simulink model "ReplayPosFilter"  (Simulink 7.8)
settings: Solver=FixedStepDiscrete  StartTime=0.0  StopTime=time(end)  FixedStep=.01  RelTol=1e-3
values from neighbouring files (symbols this model uses):
  apSampleTime = 0.01    [Load_Replay.m]    (also in loadReplayMay2013.m; loadTuneRollReplay_May2013.m; replayFlight.m)
  barAdjust = -6    [replayFlight.m]
  baroCutoff = 0.2/(2*pi)    (= 0.0318309886184)    [replayFlight.m]
  baroCutTemp = -50.0    (= -50)    [replayFlight.m]
  baroOffset = P(2)    [replayFlight.m]
  baroScale = P(1)    [replayFlight.m]
  barTGain1 = -0.0102663    [replayFlight.m]
  barTGain2 = 0.0207608    [replayFlight.m]
  barTMean1 = -161.3    [replayFlight.m]
  barTMean2 = 347.23    [replayFlight.m]
  baseHeight = GS_location(1)    [Load_Replay.m]    (also in loadReplayMay2013.m; loadTuneRollReplay_May2013.m; replayFlight.m = 225)
  baseTemp = 288.215    [GetBaroAlt.m]    (also in replayFlight.m)
  GS_location = [180 36.9898376464844 -122.051963806152]    [Load_Replay.m]    (also in loadReplayMay2013.m; loadTuneRollReplay_May2013.m; replayFlight.m = [0 36.9898376464844 -122.051963806152])
  lapseRate = -0.00198122    [replayFlight.m]
  maxDynPressure = 3000    [replayFlight.m]
  pitAdjust = -41    [replayFlight.m]
  pitCutTemp = -130.0    (= -130)    [replayFlight.m]
  pitotOffset = -1083.881038056753    (= -1083.88103806)    [replayFlight.m]
  pitotScale = 1.213292590242    (= 1.21329259024)    [replayFlight.m]
  pitTGain1 = -0.0552923    [replayFlight.m]
  pitTGain2 = -0.0950433    [replayFlight.m]
  pitTMean1 = -202.93    [replayFlight.m]
  pitTMean2 = 293.053    [replayFlight.m]
  pressureSensorCutoff = 5    [replayFlight.m]
  TData = 0.01    [Load_Replay.m]    (also in loadReplayMay2013.m; loadTuneRollReplay_May2013.m)
  Ts = apSampleTime    (= 0.01)    [Load_Replay.m]    (also in loadReplayMay2013.m; loadTuneRollReplay_May2013.m)
undefined symbols (not defined in the file or in its folder): gaind, getGSLocation, Init_onlyOnce, Init_Reset, polesd, y1, zerosd
libraries: simulink x6, aerolibconvert2 x2, SLUGS_Library x2, dsPICdrivers x1
(part 1 of 2)
settings Model: Creator=Administrator  LastModifiedBy=User
settings OptimizationCC: InitFltsAndDblsToZero=on
settings DebuggingCC: SaveWithParameterizedLinksMsg=none  FcnCallInpInsideContextMsg=Use local settings  StrictBusMsg=Warning
settings SFSimCC: SimParseCustomCode=off
settings GRTTargetCC: TargetFcnLib=ansi_tfl_tmw.mat

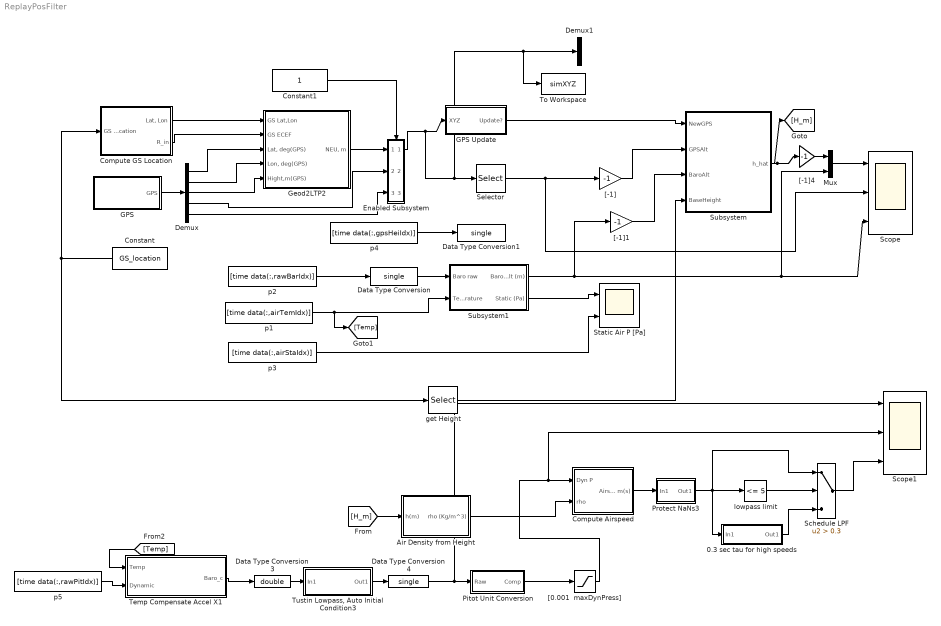
== system ReplayPosFilter ==
  " 0.3 sec tau for high speeds" : Subsystem  mask(Tustin1stOrderLowpassAutoInitialCondition){f=1, T=apSampleTime}
      mask prompts: f "Lowpass Frequency"; T "Sample Time"
      mask help: Takes a 3db rolloff frequency (in Hz, NOT radians/s) and a sample time. Performs a symbolic Tustin conversion and implements in a discrete filter. The initial output of the filter is set by the first sample.
      mask Help: Enter the desired 3db rolloff frequency in Hz and the sample time. Initial conditions are sampled automatically.
      mask Display: fprintf('%.2f Hz lowpass',f)
  Air Density from Height : Subsystem  AncestorBlock=SLUGS_Library/Air Density from Height
  Compute Airspeed : Subsystem  AncestorBlock=SLUGS_Library/Compute Airspeed
  Compute GS Location : Subsystem
  Constant : Constant  Value=GS_location  OutDataTypeStr=single
  Constant1 : Constant  OutDataTypeStr=single
  Data Type Conversion : DataTypeConversion  OutDataTypeStr=single
  Data Type Conversion1 : DataTypeConversion  OutDataTypeStr=single
  Data Type Conversion3 : DataTypeConversion  OutDataTypeStr=double
  Data Type Conversion4 : DataTypeConversion  OutDataTypeStr=single
  Demux : Demux  Outputs=5
  Demux1 : Demux  Outputs=3
  Enabled Subsystem : Subsystem  TreatAsAtomicUnit=on
  GPS : Subsystem
  GPS Update : Subsystem  mask{T=0.01}
      mask prompts: T "Sample Time"
  Geod2LTP2 : Subsystem
      mask Description:
      | This block provides transformation of the Geodetic coordinates
      | to the LTP coorinate system. The block uses two consecutive transformations
      | (Geodetic -> ECEF ->LTP).
      | Geodetic coordinates of the LTP origin should also be predetermined.
      mask Help: Oops!
      mask Display: plot(0,0,100,100,[45,40,35,40,40],[85,95,85,95,40],[85,95,85,95,40],[35,40,45,40,40],[60,40,10,20,10,14],[70,40,10,13,10,20],[56,45],[70,70],[60,60],[50,60],[60,60],[30,40],[50,60],[20,20],[30,40],[20,20],[45,55],[35,25],[75,65],[35,25])
  Mux : Mux  Inputs=2
  Pitot Unit Conversion : Subsystem  mask{bias=pitotOffset, gains=pitotScale}
      mask prompts: bias "Initial Bias"; gains "Initial Gains"
      mask help: Convert Analog readings to units
  Protect NaNs3 : Subsystem
  Schedule LPF : Switch  Criteria=u2 > Threshold  Threshold=0.3
  Scope : Scope  NumInputPorts=3
      settings: TimeRange=1400  YMin=-50~-20~-50  YMax=200~100~200
  Scope1 : Scope  NumInputPorts=3
      settings: TimeRange=1129.74  YMin=825~400~26  YMax=1175~950~38  SaveName=ScopeData2
  Selector : Selector  InputPortWidth=3  IndexOptions=Index vector (dialog)  Indices=[3]  OutputSizes=1
  Static Air P [Pa] : Scope  NumInputPorts=2
      settings: YMin=98700~98550  YMax=99500~99300
  Subsystem : Subsystem
  Subsystem1 : Subsystem
  Temp Compensate Accel X1 : Subsystem
  To Workspace : ToWorkspace  VariableName=simXYZ  SampleTime=-1  SaveFormat=Array
  "Tustin Lowpass, Auto Initial Condition3" : Subsystem  mask(Tustin1stOrderLowpassAutoInitialCondition){f=pressureSensorCutoff, T=apSampleTime}
      mask prompts: f "Lowpass Frequency"; T "Sample Time"
      mask help: Takes a 3db rolloff frequency (in Hz, NOT radians/s) and a sample time. Performs a symbolic Tustin conversion and implements in a discrete filter. The initial output of the filter is set by the first sample.
      mask Help: Enter the desired 3db rolloff frequency in Hz and the sample time. Initial conditions are sampled automatically.
      mask Display: fprintf('%.2f Hz lowpass',f)
  "[-1]" : Gain  Gain=-1
  "[-1]1" : Gain  Gain=-1
  "[-1]4" : Gain  Gain=-1
  "[0.001  maxDynPress]" : Saturate  UpperLimit=maxDynPressure  LowerLimit=0.001
  get Height : Selector  InputPortWidth=3  IndexOptions=Index vector (dialog)  Indices=[1]  OutputSizes=1
  lowpass limit : simulink/Logic and Bit Operations/Compare To Constant  relop=<=  const=5  OutDataTypeStr=uint8  ZeroCross=off
  p1 : FromWorkspace  VariableName=[time data(:,airTemIdx)]  SampleTime=apSampleTime  OutputAfterFinalValue=Setting to zero
  p2 : FromWorkspace  VariableName=[time data(:,rawBarIdx)]  SampleTime=apSampleTime  OutputAfterFinalValue=Setting to zero
  p3 : FromWorkspace  VariableName=[time data(:,airStaIdx)]  SampleTime=apSampleTime  OutputAfterFinalValue=Setting to zero
  p4 : FromWorkspace  VariableName=[time data(:,gpsHeiIdx)]  SampleTime=TData  OutputAfterFinalValue=Setting to zero
  p5 : FromWorkspace  VariableName=[time data(:,rawPitIdx)]  SampleTime=apSampleTime  OutputAfterFinalValue=Setting to zero
  wires:
  Constant/1 -> Compute GS Location/1(GS Location), get Height/1
  Demux/1 -> Geod2LTP2/3("Lat, deg(GPS)")
  Demux/2 -> Geod2LTP2/4("Lon, deg(GPS)")
  Demux/3 -> Geod2LTP2/5(Hight,m(GPS))
  Compute GS Location/2(R_in) -> Geod2LTP2/2(GS ECEF)
  Compute GS Location/1("Lat, Lon") -> Geod2LTP2/1(GS Lat,Lon)
  GPS Update/1(Update?) -> Subsystem/1(NewGPS)
  Constant1/1 -> Enabled Subsystem/Enable
  Enabled Subsystem/1(Out1) -> GPS Update/1(XYZ), Selector/1, Demux1/1, To Workspace/1
  Geod2LTP2/1("NEU, m") -> Enabled Subsystem/1(In1)
  Demux/4 -> Enabled Subsystem/2(In2)
  Demux/5 -> Enabled Subsystem/3(In3)
  "[-1]"/1 -> Subsystem/2(GPSAlt)
  GPS/1(GPS) -> Demux/1
  get Height/1 -> Subsystem/4(BaseHeight)
  p1/1 -> Subsystem1/2(Temperature), [Temp]
  Subsystem1/2(Static (Pa)) -> Static Air P [Pa]/1
  p2/1 -> Data Type Conversion/1
  Data Type Conversion/1 -> Subsystem1/1(Baro raw)
  p3/1 -> Static Air P [Pa]/2
  p4/1 -> Data Type Conversion1/1
  Subsystem/1(h_hat) -> "[-1]4"/1, [H_m]
  Selector/1 -> "[-1]"/1, Scope/2
  Subsystem1/1(Baro Alt (m)) -> "[-1]1"/1, Scope/3, Mux/2
  "[-1]1"/1 -> Subsystem/3(BaroAlt)
  Mux/1 -> Scope/1
  "[-1]4"/1 -> Mux/1
  [H_m] -> Air Density from Height/1(h(m))
  Air Density from Height/1(rho (Kg/m^3)) -> Compute Airspeed/2(rho)
  Compute Airspeed/1(Airspeed m(s)) -> Protect NaNs3/1(In1)
  lowpass limit/1 -> Schedule LPF/2
  " 0.3 sec tau for high speeds"/1(Out1) -> Schedule LPF/3
  Protect NaNs3/1(Out1) -> " 0.3 sec tau for high speeds"/1(In1), lowpass limit/1, Schedule LPF/1
  Data Type Conversion3/1 -> "Tustin Lowpass, Auto Initial Condition3"/1(In1)
  "Tustin Lowpass, Auto Initial Condition3"/1(Out1) -> Data Type Conversion4/1
  Data Type Conversion4/1 -> Pitot Unit Conversion/1(Raw), Scope1/1
  Pitot Unit Conversion/1(Comp) -> "[0.001  maxDynPress]"/1
  [Temp] -> Temp Compensate Accel X1/1(Temp)
  p5/1 -> Temp Compensate Accel X1/2(Dynamic)
  Temp Compensate Accel X1/1(Baro_c) -> Data Type Conversion3/1
  "[0.001  maxDynPress]"/1 -> Compute Airspeed/1(Dyn P), Scope1/2
  Schedule LPF/1 -> Scope1/3

== system ReplayPosFilter/ 0.3 sec tau for high speeds ==
  In1 : Inport
  Constant : Constant  Value=T
  Constant1 : Constant  Value=f
  Embedded MATLAB Function : MATLAB Function  TreatAsAtomicUnit=on
  Out1 : Outport
  wires:
  Constant/1 -> Embedded MATLAB Function/2(T)
  Constant1/1 -> Embedded MATLAB Function/3(f)
  Embedded MATLAB Function/1(y) -> Out1/1
  In1/1 -> Embedded MATLAB Function/1(u)

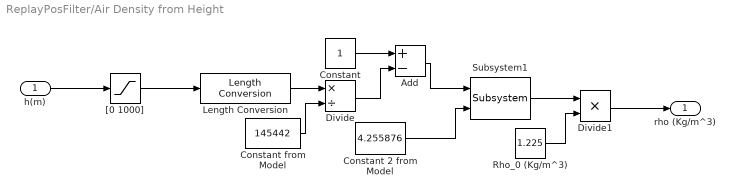
== system ReplayPosFilter/Air Density from Height ==
  h(m) : Inport
  Add : Sum  Inputs=+-
  Constant : Constant  OutDataTypeStr=single
  Constant 2 from Model : Constant  Value=4.255876  OutDataTypeStr=single
  Constant from Model : Constant  Value=145442  OutDataTypeStr=single
  Divide : Product  Inputs=*/
  Divide1 : Product
  Length Conversion : aerolibconvert2/Length Conversion  IU=m  OU=ft
  Rho_0 (Kg/m^3) : Constant  Value=1.225  OutDataTypeStr=single
  Subsystem1 : SLUGS_Library/Subsystem
  "[0 1000]" : Saturate  UpperLimit=1000  LowerLimit=0
  rho (Kg/m^3) : Outport
  wires:
  Constant/1 -> Add/1
  Divide/1 -> Add/2
  h(m)/1 -> "[0 1000]"/1
  Constant from Model/1 -> Divide/2
  Rho_0 (Kg/m^3)/1 -> Divide1/2
  Divide1/1 -> rho (Kg/m^3)/1
  Length Conversion/1 -> Divide/1
  Add/1 -> Subsystem1/1
  Constant 2 from Model/1 -> Subsystem1/2
  Subsystem1/1 -> Divide1/1
  "[0 1000]"/1 -> Length Conversion/1

== system ReplayPosFilter/Compute Airspeed ==
  Dyn P : Inport
  rho : Inport  Port=2
  Data Type Conversion1 : DataTypeConversion  OutDataTypeStr=single
  Divide2 : Product  Inputs=**/
  Subsystem2 : SLUGS_Library/Subsystem1
  "[ 0.01 50000]" : Saturate  UpperLimit=50000  LowerLimit=0.01
  a : Constant  Value=2  OutDataTypeStr=single
  Airspeed m(s) : Outport
  wires:
  "[ 0.01 50000]"/1 -> Divide2/3
  rho/1 -> "[ 0.01 50000]"/1
  Dyn P/1 -> Divide2/2
  a/1 -> Divide2/1
  Subsystem2/1 -> Airspeed m(s)/1
  Divide2/1 -> Data Type Conversion1/1
  Data Type Conversion1/1 -> Subsystem2/1

== system ReplayPosFilter/Compute GS Location ==
  GS Location : Inport
  Demux : Demux  Outputs=3
  Geod2ECEF1 : Subsystem  mask{Re=6378137, Rp=6356752.3142}
      mask prompts: Re "Enter equatorial radius, m"; Rp "Enter polar radius,m"
  Mux1 : Mux  Inputs=2
  Mux2 : Mux  Inputs=3
  "Lat, Lon" : Outport
  R_in : Outport  Port=2
  wires:
  Geod2ECEF1/3("Ze, m ") -> Mux2/3
  Geod2ECEF1/1("Xe, m ") -> Mux2/1
  Geod2ECEF1/2("Ye, m ") -> Mux2/2
  Demux/1 -> Geod2ECEF1/1("height, m")
  Demux/2 -> Mux1/2, Geod2ECEF1/2("lat, deg")
  Demux/3 -> Mux1/1, Geod2ECEF1/3(lon,deg)
  GS Location/1 -> Demux/1
  Mux1/1 -> "Lat, Lon"/1
  Mux2/1 -> R_in/1  "R_in"

== system ReplayPosFilter/Enabled Subsystem ==
  In1 : Inport
  In2 : Inport  Port=2
  In3 : Inport  Port=3
  Enable : EnablePort
  Out1 : Outport
  Out2 : Outport  Port=2
  Out3 : Outport  Port=3
  wires:
  In1/1 -> Out1/1
  In2/1 -> Out2/1
  In3/1 -> Out3/1

== system ReplayPosFilter/GPS ==
  Data Type Conversion : DataTypeConversion  OutDataTypeStr=single
  Mux : Mux  Inputs=5
  p : FromWorkspace  VariableName=[time data(:,gpsLatIdx)]  SampleTime=TData  OutputAfterFinalValue=Setting to zero
  p1 : FromWorkspace  VariableName=[time data(:,gpsLonIdx)]  SampleTime=TData  OutputAfterFinalValue=Setting to zero
  p2 : FromWorkspace  VariableName=[time data(:,gpsHeiIdx)]  SampleTime=TData  OutputAfterFinalValue=Setting to zero
  p3 : FromWorkspace  VariableName=[time data(:,gpsSogIdx)]  SampleTime=Ts  OutputAfterFinalValue=Setting to zero
  p4 : FromWorkspace  VariableName=[time data(:,gpsCogIdx)]  SampleTime=TData  OutputAfterFinalValue=Setting to zero
  GPS : Outport
  wires:
  p/1 -> Mux/1
  p1/1 -> Mux/2
  p2/1 -> Mux/3
  Mux/1 -> Data Type Conversion/1
  p3/1 -> Mux/4
  p4/1 -> Mux/5
  Data Type Conversion/1 -> GPS/1

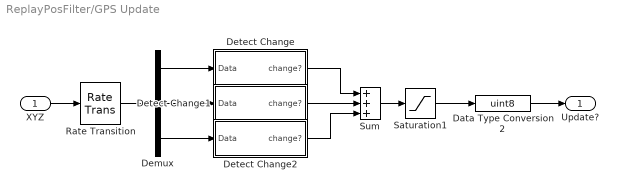
== system ReplayPosFilter/GPS Update ==
  XYZ : Inport
  Data Type Conversion2 : DataTypeConversion  OutDataTypeStr=uint8
  Demux : Demux  Outputs=3
  Detect Change : Subsystem
  Detect Change1 : Subsystem
  Detect Change2 : Subsystem
  Rate Transition : RateTransition  OutPortSampleTime=T
  Saturation1 : Saturate  UpperLimit=1  LowerLimit=0  SampleTime=T
  Sum : Sum  Inputs=3
  Update? : Outport
  wires:
  Demux/1 -> Detect Change/1(Data)
  Demux/2 -> Detect Change1/1(Data)
  Demux/3 -> Detect Change2/1(Data)
  Detect Change/1(change?) -> Sum/1
  Detect Change1/1(change?) -> Sum/2
  Detect Change2/1(change?) -> Sum/3
  Sum/1 -> Saturation1/1
  XYZ/1 -> Rate Transition/1
  Saturation1/1 -> Data Type Conversion2/1
  Rate Transition/1 -> Demux/1
  Data Type Conversion2/1 -> Update?/1

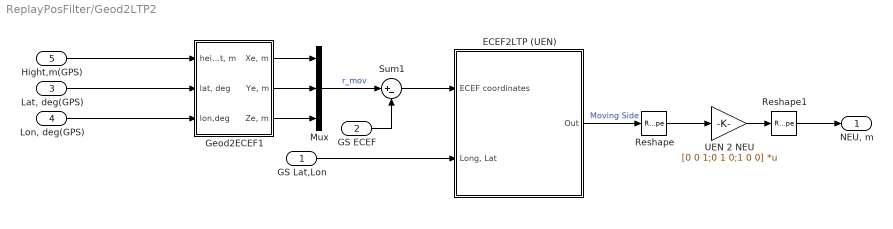
== system ReplayPosFilter/Geod2LTP2 ==
  GS Lat,Lon : Inport
  GS ECEF : Inport  Port=2
  "Lat, deg(GPS)" : Inport  Port=3
  "Lon, deg(GPS)" : Inport  Port=4
  Hight,m(GPS) : Inport  Port=5
  ECEF2LTP (UEN) : Subsystem
      mask Display: plot(0,0,100,100,[45,40,35,40,40],[85,95,85,95,40],[85,95,85,95,40],[35,40,45,40,40],[60,40,10,20,10,14],[70,40,10,13,10,20],[56,45],[70,70],[60,60],[50,60],[60,60],[30,40],[50,60],[20,20],[30,40],[20,20],[45,55],[35,25],[75,65],[35,25])
  Geod2ECEF1 : Subsystem  mask{Re=6378137, Rp=6356752.3142}
      mask prompts: Re "Enter equatorial radius, m"; Rp "Enter polar radius,m"
  Mux : Mux  Inputs=3
  Reshape : Reshape  OutputDimensionality=Column vector (2-D)
  Reshape1 : Reshape
  Sum1 : Sum  Inputs=|+-  OutDataTypeStr=single  SaturateOnIntegerOverflow=on
  UEN 2 NEU : Gain  Gain=[0 0 1;0 1 0;1 0 0]  Multiplication=Matrix(K*u)  OutDataTypeStr=float('single')  SaturateOnIntegerOverflow=on  ParamDataTypeStr=Inherit: Same as input
  "NEU, m" : Outport
  wires:
  Reshape1/1 -> "NEU, m"/1
  Reshape/1 -> UEN 2 NEU/1
  Sum1/1 -> ECEF2LTP (UEN)/1(ECEF coordinates)
  Mux/1 -> Sum1/1  "r_mov"
  Hight,m(GPS)/1 -> Geod2ECEF1/1("height, m")
  ECEF2LTP (UEN)/1(Out) -> Reshape/1  "Moving Side"
  GS ECEF/1 -> Sum1/2
  GS Lat,Lon/1 -> ECEF2LTP (UEN)/2("Long, Lat")
  "Lon, deg(GPS)"/1 -> Geod2ECEF1/3(lon,deg)
  "Lat, deg(GPS)"/1 -> Geod2ECEF1/2("lat, deg")
  Geod2ECEF1/2("Ye, m ") -> Mux/2
  Geod2ECEF1/1("Xe, m ") -> Mux/1
  Geod2ECEF1/3("Ze, m ") -> Mux/3
  UEN 2 NEU/1 -> Reshape1/1

== system ReplayPosFilter/Pitot Unit Conversion ==
  Raw : Inport
  Bias : Constant  Value=bias  OutDataTypeStr=single
  Divide : Product  OutDataTypeStr=single
  Gains : Constant  Value=gains  OutDataTypeStr=single
  Sum : Sum  Inputs=|++  OutDataTypeStr=single
  Comp : Outport
  wires:
  Bias/1 -> Sum/2
  Gains/1 -> Divide/1
  Raw/1 -> Divide/2
  Divide/1 -> Sum/1
  Sum/1 -> Comp/1

== system ReplayPosFilter/Protect NaNs3 ==
  In1 : Inport
  Integer Delay3 : Delay  DelayLength=1  InputProcessing=Inherited  SampleTime=apSampleTime
  Relational Operator2 : RelationalOperator  Operator===  OutDataTypeStr=uint(8)
  Switch3 : Switch  Criteria=u2 > Threshold  Threshold=0.3  SampleTime=.01
  Out1 : Outport
  wires:
  Integer Delay3/1 -> Switch3/3
  Switch3/1 -> Out1/1, Integer Delay3/1
  In1/1 -> Relational Operator2/2, Relational Operator2/1, Switch3/1
  Relational Operator2/1 -> Switch3/2

== system ReplayPosFilter/Subsystem ==
  NewGPS : Inport
  GPSAlt : Inport  Port=2
  BaroAlt : Inport  Port=3
  BaseHeight : Inport  Port=4
  2 FIlter Blend1 : Subsystem
  h_hat : Outport
  wires:
  2 FIlter Blend1/1(Blend) -> h_hat/1
  NewGPS/1 -> 2 FIlter Blend1/3(New GPS)
  GPSAlt/1 -> 2 FIlter Blend1/1(HiPass)
  BaroAlt/1 -> 2 FIlter Blend1/2(LoPass1)
  BaseHeight/1 -> 2 FIlter Blend1/4(baseHeight)

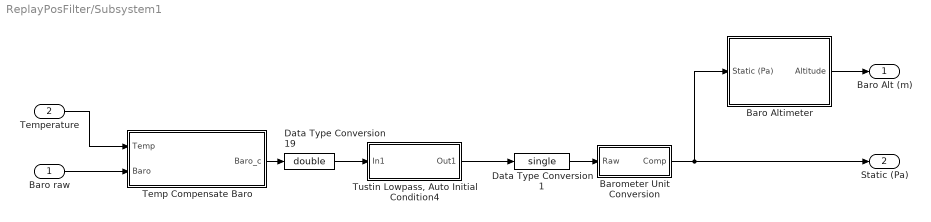
== system ReplayPosFilter/Subsystem1 ==
  Baro raw : Inport
  Temperature : Inport  Port=2
  Baro Altimeter : Subsystem
  Barometer Unit Conversion : Subsystem  mask{bias=baroOffset, gains=baroScale}
      mask prompts: bias "Initial Bias"; gains "Initial Gains"
      mask help: Convert Analog readings to units
  Data Type Conversion1 : DataTypeConversion  OutDataTypeStr=single
  Data Type Conversion19 : DataTypeConversion  OutDataTypeStr=double
  Temp Compensate Baro : Subsystem
  "Tustin Lowpass, Auto Initial Condition4" : Subsystem  mask(Tustin1stOrderLowpassAutoInitialCondition){f=pressureSensorCutoff, T=apSampleTime}
      mask prompts: f "Lowpass Frequency"; T "Sample Time"
      mask help: Takes a 3db rolloff frequency (in Hz, NOT radians/s) and a sample time. Performs a symbolic Tustin conversion and implements in a discrete filter. The initial output of the filter is set by the first sample.
      mask Help: Enter the desired 3db rolloff frequency in Hz and the sample time. Initial conditions are sampled automatically.
      mask Display: fprintf('%.2f Hz lowpass',f)
  Baro Alt (m) : Outport
  Static (Pa) : Outport  Port=2
  wires:
  Data Type Conversion19/1 -> "Tustin Lowpass, Auto Initial Condition4"/1(In1)
  Barometer Unit Conversion/1(Comp) -> Static (Pa)/1, Baro Altimeter/1(Static (Pa))
  "Tustin Lowpass, Auto Initial Condition4"/1(Out1) -> Data Type Conversion1/1
  Data Type Conversion1/1 -> Barometer Unit Conversion/1(Raw)
  Baro Altimeter/1(Altitude) -> Baro Alt (m)/1
  Temperature/1 -> Temp Compensate Baro/1(Temp)
  Temp Compensate Baro/1(Baro_c) -> Data Type Conversion19/1
  Baro raw/1 -> Temp Compensate Baro/2(Baro)

== system ReplayPosFilter/Temp Compensate Accel X1 ==
  Temp : Inport
  Dynamic : Inport  Port=2
  Compare To Constant : simulink/Logic and Bit Operations/Compare To Constant  relop=<  const=pitCutTemp  OutDataTypeStr=uint8  ZeroCross=off
  Display : Display
  Display2 : Display
  Hi Temp Compensation2 : Subsystem  mask{alpha=pitTGain2, tempMean=pitTMean2}
      mask prompts: alpha "Tempearature Coeficient (K_t)"; tempMean "Calibration Temperature Mean (T_avg)"
      mask help:
      | This block implements a temperature compensation. It implmements the following equation:
      |
      | M_tc = M_raw - K_t(T - T_avg)
  Lo Temp Compensation : Subsystem  mask{alpha=pitTGain1, tempMean=pitTMean1}
      mask prompts: alpha "Tempearature Coeficient (K_t)"; tempMean "Calibration Temperature Mean (T_avg)"
      mask help:
      | This block implements a temperature compensation. It implmements the following equation:
      |
      | M_tc = M_raw - K_t(T - T_avg)
  Logical Operator : Logic  Operator=NOT  AllPortsSameDT=off  OutDataTypeStr=boolean
  Merge : Merge
  Baro_c : Outport
  wires:
  Hi Temp Compensation2/1(Comp) -> Merge/1
  Logical Operator/1 -> Hi Temp Compensation2/Enable, Display2/1
  Merge/1 -> Baro_c/1, Display/1
  Dynamic/1 -> Lo Temp Compensation/1(Raw), Hi Temp Compensation2/1(Raw)
  Temp/1 -> Compare To Constant/1, Lo Temp Compensation/2(Temp Raw), Hi Temp Compensation2/2(Temp Raw)
  Compare To Constant/1 -> Lo Temp Compensation/Enable, Logical Operator/1
  Lo Temp Compensation/1(Comp) -> Merge/2

== system ReplayPosFilter/Tustin Lowpass, Auto Initial Condition3 ==
  In1 : Inport
  Constant : Constant  Value=T
  Constant1 : Constant  Value=f
  Embedded MATLAB Function : MATLAB Function  TreatAsAtomicUnit=on
  Out1 : Outport
  wires:
  Constant/1 -> Embedded MATLAB Function/2(T)
  Constant1/1 -> Embedded MATLAB Function/3(f)
  Embedded MATLAB Function/1(y) -> Out1/1
  In1/1 -> Embedded MATLAB Function/1(u)

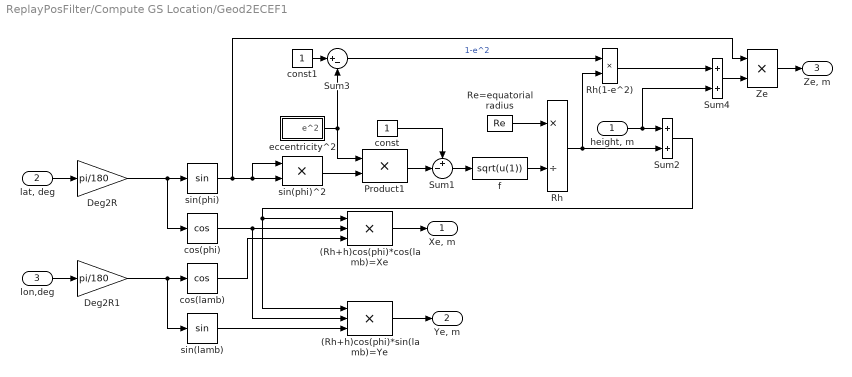
== system ReplayPosFilter/Compute GS Location/Geod2ECEF1 ==
  "height, m" : Inport
  "lat, deg" : Inport  Port=2
  lon,deg : Inport  Port=3
  (Rh+h)cos(phi)*cos(lamb)=Xe : Product  Inputs=3  OutDataTypeStr=single  SaturateOnIntegerOverflow=on  InputSameDT=on
  (Rh+h)cos(phi)*sin(lamb)=Ye : Product  Inputs=3  OutDataTypeStr=single  SaturateOnIntegerOverflow=on  InputSameDT=on
  Deg2R : Gain  Gain=pi/180  OutDataTypeStr=float('single')  SaturateOnIntegerOverflow=on  ParamDataTypeStr=Inherit: Same as input
  Deg2R1 : Gain  Gain=pi/180  OutDataTypeStr=float('single')  SaturateOnIntegerOverflow=on  ParamDataTypeStr=Inherit: Same as input
  Product1 : Product  SaturateOnIntegerOverflow=on  InputSameDT=on  OutDataTypeStr=Inherit: Same as first input
  Re=equatorial radius : Constant  Value=Re  OutDataTypeStr=single
  Rh : Product  Inputs=*/  OutDataTypeStr=single  SaturateOnIntegerOverflow=on  InputSameDT=on
  Rh(1-e^2) : Product  OutDataTypeStr=single  SaturateOnIntegerOverflow=on  InputSameDT=on
  Sum1 : Sum  Inputs=+-|  SaturateOnIntegerOverflow=on  InputSameDT=on  OutDataTypeStr=Inherit: Same as first input
  Sum2 : Sum  SaturateOnIntegerOverflow=on  InputSameDT=on  OutDataTypeStr=Inherit: Same as first input
      settings: AttributesFormatString=Rh+h
  Sum3 : Sum  Inputs=|+-  SaturateOnIntegerOverflow=on  InputSameDT=on  OutDataTypeStr=Inherit: Same as first input
  Sum4 : Sum  OutDataTypeStr=single  SaturateOnIntegerOverflow=on  InputSameDT=on
      settings: AttributesFormatString=(1-e^2)Rh+h
  Ze : Product  OutDataTypeStr=single  SaturateOnIntegerOverflow=on  InputSameDT=on
  const : Constant  OutDataTypeStr=single
  const1 : Constant  OutDataTypeStr=single
  cos(lamb) : Trigonometry  Operator=cos
  cos(phi) : Trigonometry  Operator=cos
  eccentricity^2 : Subsystem
  f : Fcn  Expr=sqrt(u(1))
  sin(lamb) : Trigonometry
  sin(phi) : Trigonometry
  sin(phi)^2 : Product  SaturateOnIntegerOverflow=on  InputSameDT=on  OutDataTypeStr=Inherit: Same as first input
  "Xe, m " : Outport
  "Ye, m " : Outport  Port=2
  "Ze, m " : Outport  Port=3
  wires:
  (Rh+h)cos(phi)*sin(lamb)=Ye/1 -> "Ye, m "/1
  (Rh+h)cos(phi)*cos(lamb)=Xe/1 -> "Xe, m "/1
  Sum2/1 -> (Rh+h)cos(phi)*cos(lamb)=Xe/1, (Rh+h)cos(phi)*sin(lamb)=Ye/1
  Deg2R1/1 -> sin(lamb)/1, cos(lamb)/1
  Deg2R/1 -> sin(phi)/1, cos(phi)/1
  Ze/1 -> "Ze, m "/1
  sin(lamb)/1 -> (Rh+h)cos(phi)*sin(lamb)=Ye/3
  cos(lamb)/1 -> (Rh+h)cos(phi)*cos(lamb)=Xe/3
  cos(phi)/1 -> (Rh+h)cos(phi)*sin(lamb)=Ye/2, (Rh+h)cos(phi)*cos(lamb)=Xe/2
  lon,deg/1 -> Deg2R1/1
  Sum4/1 -> Ze/2
  Rh(1-e^2)/1 -> Sum4/1
  Sum3/1 -> Rh(1-e^2)/1  "1-e^2"
  const1/1 -> Sum3/1
  sin(phi)^2/1 -> Product1/2
  eccentricity^2/1(e^2) -> Sum3/2, Product1/1
  "height, m"/1 -> Sum2/1, Sum4/2
  const/1 -> Sum1/1
  Sum1/1 -> f/1
  Product1/1 -> Sum1/2
  Rh/1 -> Rh(1-e^2)/2, Sum2/2
  Re=equatorial radius/1 -> Rh/1
  f/1 -> Rh/2
  sin(phi)/1 -> Ze/1, sin(phi)^2/2, sin(phi)^2/1
  "lat, deg"/1 -> Deg2R/1

== system ReplayPosFilter/GPS Update/Detect Change ==
  Data : Inport
  Abs1 : Abs  SampleTime=T
  Difference1 : simulink/Discrete/Difference  ICPrevInput=0.0  InputProcessing=Inherited  OutMin=[]  OutMax=[]  OutDataType=sfix(16)  OutScaling=2^-10  DoSatur=off
  Saturation1 : Saturate  UpperLimit=1  LowerLimit=0  SampleTime=T
  change? : Outport
  wires:
  Difference1/1 -> Abs1/1
  Abs1/1 -> Saturation1/1
  Data/1 -> Difference1/1
  Saturation1/1 -> change?/1

== system ReplayPosFilter/GPS Update/Detect Change1 ==
  Data : Inport
  Abs1 : Abs  SampleTime=T
  Difference1 : simulink/Discrete/Difference  ICPrevInput=0.0  InputProcessing=Inherited  OutMin=[]  OutMax=[]  OutDataType=sfix(16)  OutScaling=2^-10  DoSatur=off
  Saturation1 : Saturate  UpperLimit=1  LowerLimit=0  SampleTime=T
  change? : Outport
  wires:
  Saturation1/1 -> change?/1
  Data/1 -> Difference1/1
  Abs1/1 -> Saturation1/1
  Difference1/1 -> Abs1/1

== system ReplayPosFilter/GPS Update/Detect Change2 ==
  Data : Inport
  Abs1 : Abs  SampleTime=T
  Difference1 : simulink/Discrete/Difference  ICPrevInput=0.0  InputProcessing=Inherited  OutMin=[]  OutMax=[]  OutDataType=sfix(16)  OutScaling=2^-10  DoSatur=off
  Saturation1 : Saturate  UpperLimit=1  LowerLimit=0  SampleTime=T
  change? : Outport
  wires:
  Difference1/1 -> Abs1/1
  Abs1/1 -> Saturation1/1
  Data/1 -> Difference1/1
  Saturation1/1 -> change?/1

== system ReplayPosFilter/Geod2LTP2/ECEF2LTP (UEN) ==
  ECEF coordinates : Inport
  "Long, Lat" : Inport  Port=2
  Deg2R : Gain  Gain=pi/180  SaturateOnIntegerOverflow=on  OutDataTypeStr=Inherit: Same as input  ParamDataTypeStr=Inherit: Same as input
  Demux3 : Demux  Outputs=2
  From Body to Universal1 : Subsystem
  Product1 : Product  Multiplication=Matrix(*)  SaturateOnIntegerOverflow=on  InputSameDT=on  OutDataTypeStr=Inherit: Same as first input
  Out : Outport
  wires:
  From Body to Universal1/1(DCM) -> Product1/1
  ECEF coordinates/1 -> Product1/2
  Deg2R/1 -> Demux3/1
  Demux3/1 -> From Body to Universal1/1(long)
  Demux3/2 -> From Body to Universal1/2(lat)
  Product1/1 -> Out/1
  "Long, Lat"/1 -> Deg2R/1

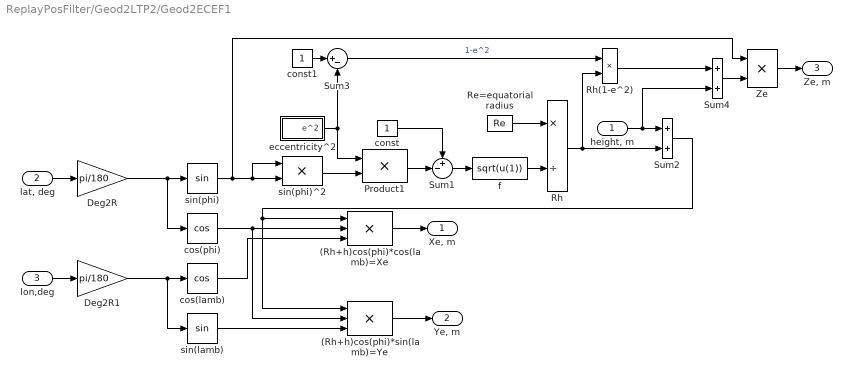
== system ReplayPosFilter/Geod2LTP2/Geod2ECEF1 ==
  "height, m" : Inport
  "lat, deg" : Inport  Port=2
  lon,deg : Inport  Port=3
  (Rh+h)cos(phi)*cos(lamb)=Xe : Product  Inputs=3  OutDataTypeStr=single  SaturateOnIntegerOverflow=on  InputSameDT=on
  (Rh+h)cos(phi)*sin(lamb)=Ye : Product  Inputs=3  OutDataTypeStr=single  SaturateOnIntegerOverflow=on  InputSameDT=on
  Deg2R : Gain  Gain=pi/180  OutDataTypeStr=float('single')  SaturateOnIntegerOverflow=on  ParamDataTypeStr=Inherit: Same as input
  Deg2R1 : Gain  Gain=pi/180  OutDataTypeStr=float('single')  SaturateOnIntegerOverflow=on  ParamDataTypeStr=Inherit: Same as input
  Product1 : Product  SaturateOnIntegerOverflow=on  InputSameDT=on  OutDataTypeStr=Inherit: Same as first input
  Re=equatorial radius : Constant  Value=Re  OutDataTypeStr=single
  Rh : Product  Inputs=*/  OutDataTypeStr=single  SaturateOnIntegerOverflow=on  InputSameDT=on
  Rh(1-e^2) : Product  OutDataTypeStr=single  SaturateOnIntegerOverflow=on  InputSameDT=on
  Sum1 : Sum  Inputs=+-|  SaturateOnIntegerOverflow=on  InputSameDT=on  OutDataTypeStr=Inherit: Same as first input
  Sum2 : Sum  SaturateOnIntegerOverflow=on  InputSameDT=on  OutDataTypeStr=Inherit: Same as first input
      settings: AttributesFormatString=Rh+h
  Sum3 : Sum  Inputs=|+-  SaturateOnIntegerOverflow=on  InputSameDT=on  OutDataTypeStr=Inherit: Same as first input
  Sum4 : Sum  OutDataTypeStr=single  SaturateOnIntegerOverflow=on  InputSameDT=on
      settings: AttributesFormatString=(1-e^2)Rh+h
  Ze : Product  OutDataTypeStr=single  SaturateOnIntegerOverflow=on  InputSameDT=on
  const : Constant  OutDataTypeStr=single
  const1 : Constant  OutDataTypeStr=single
  cos(lamb) : Trigonometry  Operator=cos
  cos(phi) : Trigonometry  Operator=cos
  eccentricity^2 : Subsystem
  f : Fcn  Expr=sqrt(u(1))
  sin(lamb) : Trigonometry
  sin(phi) : Trigonometry
  sin(phi)^2 : Product  SaturateOnIntegerOverflow=on  InputSameDT=on  OutDataTypeStr=Inherit: Same as first input
  "Xe, m " : Outport
  "Ye, m " : Outport  Port=2
  "Ze, m " : Outport  Port=3
  wires:
  (Rh+h)cos(phi)*sin(lamb)=Ye/1 -> "Ye, m "/1
  (Rh+h)cos(phi)*cos(lamb)=Xe/1 -> "Xe, m "/1
  Sum2/1 -> (Rh+h)cos(phi)*cos(lamb)=Xe/1, (Rh+h)cos(phi)*sin(lamb)=Ye/1
  Deg2R1/1 -> sin(lamb)/1, cos(lamb)/1
  Deg2R/1 -> sin(phi)/1, cos(phi)/1
  Ze/1 -> "Ze, m "/1
  sin(lamb)/1 -> (Rh+h)cos(phi)*sin(lamb)=Ye/3
  cos(lamb)/1 -> (Rh+h)cos(phi)*cos(lamb)=Xe/3
  cos(phi)/1 -> (Rh+h)cos(phi)*sin(lamb)=Ye/2, (Rh+h)cos(phi)*cos(lamb)=Xe/2
  lon,deg/1 -> Deg2R1/1
  Sum4/1 -> Ze/2
  Rh(1-e^2)/1 -> Sum4/1
  Sum3/1 -> Rh(1-e^2)/1  "1-e^2"
  const1/1 -> Sum3/1
  sin(phi)^2/1 -> Product1/2
  eccentricity^2/1(e^2) -> Sum3/2, Product1/1
  "height, m"/1 -> Sum2/1, Sum4/2
  const/1 -> Sum1/1
  Sum1/1 -> f/1
  Product1/1 -> Sum1/2
  Rh/1 -> Rh(1-e^2)/2, Sum2/2
  Re=equatorial radius/1 -> Rh/1
  f/1 -> Rh/2
  sin(phi)/1 -> Ze/1, sin(phi)^2/2, sin(phi)^2/1
  "lat, deg"/1 -> Deg2R/1

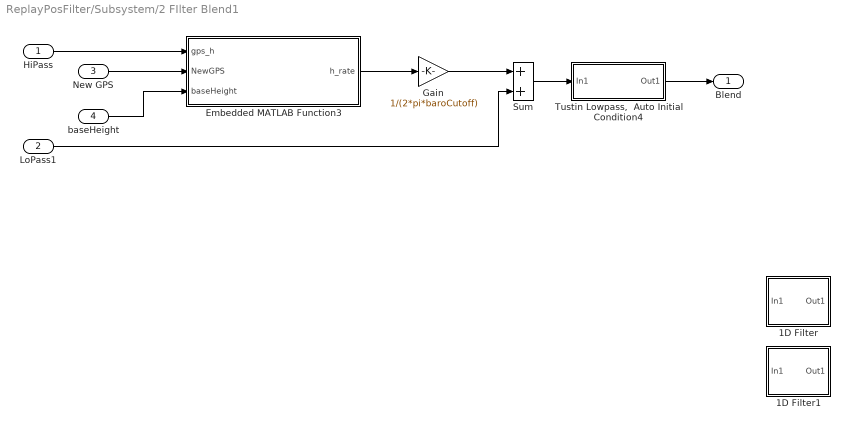
== system ReplayPosFilter/Subsystem/2 FIlter Blend1 ==
  HiPass : Inport
  LoPass1 : Inport  Port=2
  New GPS : Inport  Port=3
  baseHeight : Inport  Port=4
  1D Filter : Subsystem  AncestorBlock=SLUGS_Library/Singnal Routing & Conditioning/3D Filter  RTWFcnName=TustinFilter3D  mask{zval=[], pval=-baroCutoff, kval=1, TSample=apSampleTime}
      mask prompts: zval "Zeros"; pval "Poles"; kval "Gains"; TSample "Sample Time"
      settings: RTWFcnNameOpts=User specified  RTWFileNameOpts=Use function name
      mask Display:
      | droots(zval,pval,kval)
      | port_label('input',1,'1D')
  1D Filter1 : Subsystem  AncestorBlock=SLUGS_Library/Singnal Routing & Conditioning/3D Filter  RTWFcnName=TustinFilter3D  mask{zval=[], pval=baroCutoff, kval=1, TSample=apSampleTime}
      mask prompts: zval "Zeros"; pval "Poles"; kval "Gains"; TSample "Sample Time"
      settings: RTWFcnNameOpts=User specified  RTWFileNameOpts=Use function name
      mask Display:
      | droots(zval,pval,kval)
      | port_label('input',1,'1D')
  Embedded MATLAB Function3 : MATLAB Function  TreatAsAtomicUnit=on
  Gain : Gain  Gain=1/(2*pi*baroCutoff)
  Sum : Sum  OutDataTypeStr=single
  "Tustin Lowpass,  Auto Initial Condition4" : Subsystem  mask(Tustin1stOrderLowpassAutoInitialCondition){f=baroCutoff, T=apSampleTime}
      mask prompts: f "Lowpass Frequency"; T "Sample Time"
      mask help: Takes a 3db rolloff frequency (in Hz, NOT radians/s) and a sample time. Performs a symbolic Tustin conversion and implements in a discrete filter. The initial output of the filter is set by the first sample.
      mask Help: Enter the desired 3db rolloff frequency in Hz and the sample time. Initial conditions are sampled automatically.
      mask Display: fprintf('%.2f Hz lowpass',f)
  Blend : Outport
  wires:
  Sum/1 -> "Tustin Lowpass,  Auto Initial Condition4"/1(In1)
  New GPS/1 -> Embedded MATLAB Function3/2(NewGPS)
  HiPass/1 -> Embedded MATLAB Function3/1(gps_h)
  baseHeight/1 -> Embedded MATLAB Function3/3(baseHeight)
  Embedded MATLAB Function3/1(h_rate) -> Gain/1
  "Tustin Lowpass,  Auto Initial Condition4"/1(Out1) -> Blend/1
  Gain/1 -> Sum/1
  LoPass1/1 -> Sum/2

== system ReplayPosFilter/Subsystem1/Baro Altimeter ==
  Static (Pa) : Inport
  Compute Barometric Height : Subsystem  mask{baseTemp=baseTemp, LapseRate=lapseRate}
      mask prompts: baseTemp "Base Station Temperature (K)"; LapseRate "Lapse Rate (C/ft)"
      mask help:
      | Produces Altitude in meters from Barometric Pressure in Pascals. Altitude is valid from MSL to 6000 ft.
      |
      | The method implemented here was developed by Ren Curry
  Enabled Subsystem : Subsystem  TreatAsAtomicUnit=on
  Enables/Disables the Computation of  initial Baro Bias : MATLAB Function  TreatAsAtomicUnit=on
  GS Height : Subsystem
  Initial Baro Bias : Subsystem  TreatAsAtomicUnit=on
  Logical Operator : Logic  Operator=NOT  AllPortsSameDT=off  OutDataTypeStr=boolean
  Sum1 : Sum  Inputs=++|  OutDataTypeStr=single
  Zero Out Height : Subsystem  TreatAsAtomicUnit=on
  Altitude : Outport
  wires:
  Compute Barometric Height/1("Altitude, m") -> Zero Out Height/2(Computed Height), Sum1/2
  Static (Pa)/1 -> Initial Baro Bias/1(Baro (Pa)), Compute Barometric Height/3(Baro (Pa))
  Enables/Disables the Computation of  initial Baro Bias/1(tOut) -> Initial Baro Bias/Enable, Zero Out Height/Enable, Logical Operator/1
  GS Height/1(GS Height) -> Compute Barometric Height/1(Base Height (m)), Zero Out Height/1(Base Height)
  Initial Baro Bias/1(Baro (Gnd)) -> Compute Barometric Height/2(Base Pressure (Pa))
  Zero Out Height/1(Height Offset) -> Sum1/1
  Logical Operator/1 -> Enabled Subsystem/Enable
  Sum1/1 -> Enabled Subsystem/1(In1)
  Enabled Subsystem/1(Out1) -> Altitude/1

== system ReplayPosFilter/Subsystem1/Barometer Unit Conversion ==
  Raw : Inport
  Bias : Constant  Value=bias  OutDataTypeStr=single
  Divide : Product  OutDataTypeStr=single
  Gains : Constant  Value=gains  OutDataTypeStr=single
  Sum : Sum  Inputs=|++  OutDataTypeStr=single
  Comp : Outport
  wires:
  Bias/1 -> Sum/2
  Raw/1 -> Divide/2
  Gains/1 -> Divide/1
  Divide/1 -> Sum/1
  Sum/1 -> Comp/1

== system ReplayPosFilter/Subsystem1/Temp Compensate Baro ==
  Temp : Inport
  Baro : Inport  Port=2
  Compare To Constant : simulink/Logic and Bit Operations/Compare To Constant  relop=<  const=baroCutTemp  OutDataTypeStr=uint8  ZeroCross=off
  Hi Temp Compensation : Subsystem  mask{alpha=barTGain2, tempMean=barTMean2}
      mask prompts: alpha "Tempearature Coeficient (K_t)"; tempMean "Calibration Temperature Mean (T_avg)"
      mask help:
      | This block implements a temperature compensation. It implmements the following equation:
      |
      | M_tc = M_raw - K_t(T - T_avg)
  Lo Temp Compensation : Subsystem  mask{alpha=barTGain1, tempMean=barTMean1}
      mask prompts: alpha "Tempearature Coeficient (K_t)"; tempMean "Calibration Temperature Mean (T_avg)"
      mask help:
      | This block implements a temperature compensation. It implmements the following equation:
      |
      | M_tc = M_raw - K_t(T - T_avg)
  Logical Operator : Logic  Operator=NOT  AllPortsSameDT=off  OutDataTypeStr=boolean
  Merge : Merge
  Baro_c : Outport
  wires:
  Compare To Constant/1 -> Logical Operator/1, Lo Temp Compensation/Enable
  Temp/1 -> Compare To Constant/1, Hi Temp Compensation/2(Temp Raw), Lo Temp Compensation/2(Temp Raw)
  Baro/1 -> Hi Temp Compensation/1(Raw), Lo Temp Compensation/1(Raw)
  Lo Temp Compensation/1(Comp) -> Merge/2
  Merge/1 -> Baro_c/1
  Logical Operator/1 -> Hi Temp Compensation/Enable
  Hi Temp Compensation/1(Comp) -> Merge/1

== system ReplayPosFilter/Subsystem1/Tustin Lowpass, Auto Initial Condition4 ==
  In1 : Inport
  Constant : Constant  Value=T
  Constant1 : Constant  Value=f
  Embedded MATLAB Function : MATLAB Function  TreatAsAtomicUnit=on
  Out1 : Outport
  wires:
  In1/1 -> Embedded MATLAB Function/1(u)
  Embedded MATLAB Function/1(y) -> Out1/1
  Constant1/1 -> Embedded MATLAB Function/3(f)
  Constant/1 -> Embedded MATLAB Function/2(T)

== system ReplayPosFilter/Temp Compensate Accel X1/Hi Temp Compensation2 ==
  Raw : Inport
  Temp Raw : Inport  Port=2
  Enable : EnablePort
  Divide1 : Product  OutDataTypeStr=single
  Mean Temperature for Calibration : Constant  Value=tempMean  OutDataTypeStr=single
  Sum1 : Sum  Inputs=|+-  OutDataTypeStr=single
  Sum2 : Sum  Inputs=|+-  OutDataTypeStr=single
  gains : Constant  Value=alpha  OutDataTypeStr=single
  Comp : Outport
  wires:
  Mean Temperature for Calibration/1 -> Sum1/2
  Raw/1 -> Sum2/1
  Temp Raw/1 -> Sum1/1
  Sum1/1 -> Divide1/2
  gains/1 -> Divide1/1
  Divide1/1 -> Sum2/2
  Sum2/1 -> Comp/1

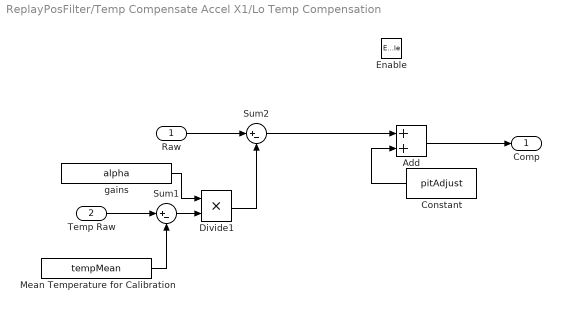
== system ReplayPosFilter/Temp Compensate Accel X1/Lo Temp Compensation ==
  Raw : Inport
  Temp Raw : Inport  Port=2
  Enable : EnablePort
  Add : Sum  OutDataTypeStr=single
  Constant : Constant  Value=pitAdjust  OutDataTypeStr=single
  Divide1 : Product  OutDataTypeStr=single
  Mean Temperature for Calibration : Constant  Value=tempMean  OutDataTypeStr=single
  Sum1 : Sum  Inputs=|+-  OutDataTypeStr=single
  Sum2 : Sum  Inputs=|+-  OutDataTypeStr=single
  gains : Constant  Value=alpha  OutDataTypeStr=single
  Comp : Outport
  wires:
  Add/1 -> Comp/1
  Constant/1 -> Add/2
  Sum2/1 -> Add/1
  Divide1/1 -> Sum2/2
  gains/1 -> Divide1/1
  Sum1/1 -> Divide1/2
  Temp Raw/1 -> Sum1/1
  Raw/1 -> Sum2/1
  Mean Temperature for Calibration/1 -> Sum1/2

== system ReplayPosFilter/Compute GS Location/Geod2ECEF1/eccentricity^2 ==
  " " : Product  OutDataTypeStr=single  SaturateOnIntegerOverflow=on  InputSameDT=on
  Re=equatorial radius1 : Constant  Value=Re  OutDataTypeStr=single
  Rp=polar radius : Constant  Value=Rp  OutDataTypeStr=single
  Sum5 : Sum  Inputs=|+-  SaturateOnIntegerOverflow=on  InputSameDT=on  OutDataTypeStr=Inherit: Same as first input
  const2 : Constant  OutDataTypeStr=single
  e^1 : Product  Inputs=*/  OutDataTypeStr=single  SaturateOnIntegerOverflow=on  InputSameDT=on
  e^2 : Outport
  wires:
  Sum5/1 -> e^2/1
  " "/1 -> Sum5/2
  e^1/1 -> " "/1, " "/2
  const2/1 -> Sum5/1
  Rp=polar radius/1 -> e^1/1
  Re=equatorial radius1/1 -> e^1/2

== system ReplayPosFilter/Geod2LTP2/ECEF2LTP (UEN)/From Body to Universal1 ==
  long : Inport
  lat : Inport  Port=2
  Mux : Mux  Inputs=2
  Reshape 9x1->3x1 : Reshape  OutputDimensionality=Customize  OutputDimensions=[3,3]
  Rotation Matrix from Long//Lat : Subsystem
      mask Type: Vector Transformation
      mask Description: Vector Transformation
      mask Display: disp('axis')
  DCM : Outport
  wires:
  Reshape 9x1->3x1/1 -> DCM/1
  Rotation Matrix from Long//Lat/1(DCM) -> Reshape 9x1->3x1/1
  Mux/1 -> Rotation Matrix from Long//Lat/1(long lat)
  long/1 -> Mux/1
  lat/1 -> Mux/2

== system ReplayPosFilter/Geod2LTP2/Geod2ECEF1/eccentricity^2 ==
  " " : Product  OutDataTypeStr=single  SaturateOnIntegerOverflow=on  InputSameDT=on
  Re=equatorial radius1 : Constant  Value=Re  OutDataTypeStr=single
  Rp=polar radius : Constant  Value=Rp  OutDataTypeStr=single
  Sum5 : Sum  Inputs=|+-  SaturateOnIntegerOverflow=on  InputSameDT=on  OutDataTypeStr=Inherit: Same as first input
  const2 : Constant  OutDataTypeStr=single
  e^1 : Product  Inputs=*/  OutDataTypeStr=single  SaturateOnIntegerOverflow=on  InputSameDT=on
  e^2 : Outport
  wires:
  Sum5/1 -> e^2/1
  " "/1 -> Sum5/2
  e^1/1 -> " "/1, " "/2
  const2/1 -> Sum5/1
  Rp=polar radius/1 -> e^1/1
  Re=equatorial radius1/1 -> e^1/2

== system ReplayPosFilter/Subsystem/2 FIlter Blend1/1D Filter ==
  In1 : Inport
  Data Type Conversion1 : DataTypeConversion  OutDataTypeStr=single
  Data Type Conversion2 : DataTypeConversion  OutDataTypeStr=double
  Filter2 : Subsystem  mask(DiscretizedZeroPole){Zeros=zval, Poles=pval, Gain=kval, AbsTol=auto, SampleTime=TSample, method=tustin, Wc=1}
      mask prompts: Zeros "Zeros (enter in s-main:)"; Poles "Poles (enter in s-domain:)"; Gain "Gain (enter in s-domain:)"; AbsTol "Absolute tolerance:"; SampleTime "Sample time:"; Wc "Critical Frequency (Hz):"
      mask help: Continuous mask uses c2d to transform parameters onto the Discrete Zero-Pole block inside.
      mask init:
      | st=SampleTime;
      | if length(st)>1
      |     st=SampleTime(1);
      | end
      | if(st>0)
      |     [zerosd,polesd,gaind] = sldiscutil('disczpk', {st,method,Wc,Zeros,Poles,Gain});
      | end	
      | s = get_param(gcb,'maskvalues');
      | zeross = s{1};
      | poless = s{2};
      | gainss = s{3};
      | %zerosc = eval(zeross);
      | %polesc = eval(poless);
      | %gainsc = eval(gainss);
      | sldiscutil('initzpkmask', st);
      | if(st==0)
      | set_param([gcb '/Zero Pole'], 'AbsoluteTolerance', AbsTol);
      | end
      mask StyleString: edit,edit,edit,edit,edit,popup(zoh|foh|tustin|prewarp|matched),edit
      mask CallbackString: |||||hidecrit|
      mask Display:
      | droots(zeross,poless,gainss)
      | text( 0.5, 1.0, method, 'verticalAlignment','top')
  Out1 : Outport
  wires:
  Data Type Conversion1/1 -> Out1/1
  Data Type Conversion2/1 -> Filter2/1(In1)
  In1/1 -> Data Type Conversion2/1
  Filter2/1(Out1) -> Data Type Conversion1/1

== system ReplayPosFilter/Subsystem/2 FIlter Blend1/1D Filter1 ==
  In1 : Inport
  Data Type Conversion1 : DataTypeConversion  OutDataTypeStr=single
  Data Type Conversion2 : DataTypeConversion  OutDataTypeStr=double
  Filter2 : Subsystem  mask(DiscretizedZeroPole){Zeros=zval, Poles=pval, Gain=kval, AbsTol=auto, SampleTime=TSample, method=tustin, Wc=1}
      mask prompts: Zeros "Zeros (enter in s-main:)"; Poles "Poles (enter in s-domain:)"; Gain "Gain (enter in s-domain:)"; AbsTol "Absolute tolerance:"; SampleTime "Sample time:"; Wc "Critical Frequency (Hz):"
      mask help: Continuous mask uses c2d to transform parameters onto the Discrete Zero-Pole block inside.
      mask init: same as ReplayPosFilter/Subsystem/2 FIlter Blend1/1D Filter/Filter2
      mask StyleString: edit,edit,edit,edit,edit,popup(zoh|foh|tustin|prewarp|matched),edit
      mask CallbackString: |||||hidecrit|
      mask Display:
      | droots(zeross,poless,gainss)
      | text( 0.5, 1.0, method, 'verticalAlignment','top')
  Out1 : Outport
  wires:
  Filter2/1(Out1) -> Data Type Conversion1/1
  In1/1 -> Data Type Conversion2/1
  Data Type Conversion2/1 -> Filter2/1(In1)
  Data Type Conversion1/1 -> Out1/1

== system ReplayPosFilter/Subsystem/2 FIlter Blend1/Tustin Lowpass,  Auto Initial Condition4 ==
  In1 : Inport
  Constant : Constant  Value=T
  Constant1 : Constant  Value=f
  Embedded MATLAB Function : MATLAB Function  TreatAsAtomicUnit=on
  Out1 : Outport
  wires:
  Constant/1 -> Embedded MATLAB Function/2(T)
  Constant1/1 -> Embedded MATLAB Function/3(f)
  Embedded MATLAB Function/1(y) -> Out1/1
  In1/1 -> Embedded MATLAB Function/1(u)

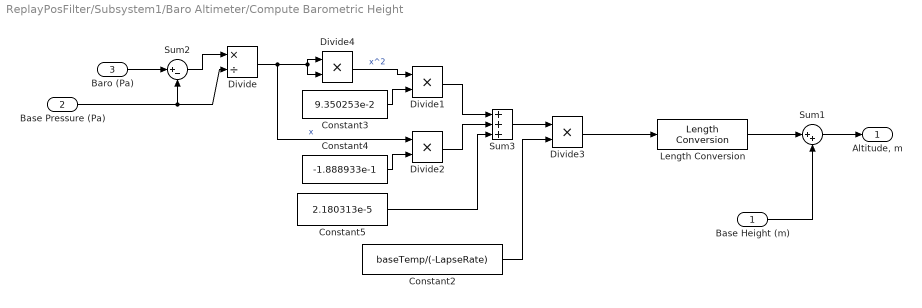
== system ReplayPosFilter/Subsystem1/Baro Altimeter/Compute Barometric Height ==
  Base Height (m) : Inport
  Base Pressure (Pa) : Inport  Port=2
  Baro (Pa) : Inport  Port=3
  Constant2 : Constant  Value=baseTemp/(-LapseRate)  OutDataTypeStr=single
  Constant3 : Constant  Value=9.350253e-2  OutDataTypeStr=single
  Constant4 : Constant  Value=-1.888933e-1  OutDataTypeStr=single
  Constant5 : Constant  Value=2.180313e-5  OutDataTypeStr=single
  Divide : Product  Inputs=*/  OutDataTypeStr=single
  Divide{1..4} (4 alike) : Product  OutDataTypeStr=single
  Length Conversion : aerolibconvert2/Length Conversion  IU=ft  OU=m
  Sum1 : Sum  Inputs=|++  OutDataTypeStr=single
  Sum2 : Sum  Inputs=|+-  OutDataTypeStr=single
  Sum3 : Sum  Inputs=3  OutDataTypeStr=single
  "Altitude, m" : Outport
  wires:
  Length Conversion/1 -> Sum1/1
  Sum2/1 -> Divide/1
  Sum1/1 -> "Altitude, m"/1
  Divide3/1 -> Length Conversion/1
  Constant2/1 -> Divide3/2
  Sum3/1 -> Divide3/1
  Constant5/1 -> Sum3/3
  Divide2/1 -> Sum3/2
  Divide1/1 -> Sum3/1
  Constant4/1 -> Divide2/2
  Constant3/1 -> Divide1/2
  Divide4/1 -> Divide1/1  "x^2"
  Divide/1 -> Divide2/1, Divide4/1, Divide4/2  "x"
  Base Pressure (Pa)/1 -> Divide/2, Sum2/2
  Base Height (m)/1 -> Sum1/2
  Baro (Pa)/1 -> Sum2/1

== system ReplayPosFilter/Subsystem1/Baro Altimeter/Enabled Subsystem ==
  In1 : Inport
  Enable : EnablePort
  Out1 : Outport  InitialOutput=baseHeight
  wires:
  In1/1 -> Out1/1

== system ReplayPosFilter/Subsystem1/Baro Altimeter/GS Height ==
  Demux : Demux  Outputs=[1 2]
  Get the GS Location [updateSensorMCUState.c] : dsPICdrivers/OTHERS/C Function Call  Tag=dsPIC_dsPIC_CFunctionCall  FctUpdate=Output Function  fctName='getGSLocation'  INPUT_SIZE=1  INPUT1=--  INPUT2=--  INPUT3=--  OUTPUT_SIZE=3  OUTPUT1=real32  SampleTime=0.01  InputType=[ ]  OutputType=[ 7 ]  FctDeclaration=extern void getGSLocation(real32_T* y1);  FctCall=getGSLocation(*%y1);  OrderingInOutPopup=None  FctStart=None  FctStart_Name=Init_onlyOnce  FctStart_Declaration=inline extern void Init_onlyOnce();  FctStart_Call=Init_onlyOnce();  FctInit=None  FctInit_Name=Init_Reset  FctInit_Declaration=inline extern void Init_Reset();  FctInit_Call=Init_Reset();  PinDigitalInput=[]  PinDigitalOutput=[]  AnalogueInput=[]
  Terminator : Terminator
  GS Height : Outport
  wires:
  Get the GS Location [updateSensorMCUState.c]/1 -> Demux/1
  Demux/2 -> Terminator/1
  Demux/1 -> GS Height/1

== system ReplayPosFilter/Subsystem1/Baro Altimeter/Initial Baro Bias ==
  Baro (Pa) : Inport
  Enable : EnablePort
  Data Type Conversion : DataTypeConversion  OutDataTypeStr=double
  Data Type Conversion1 : DataTypeConversion  OutDataTypeStr=single
  Low Pass8 : Subsystem  mask(DiscretizedZeroPole){Zeros=[], Poles=[-3], Gain=3, AbsTol=auto, SampleTime=.01, method=tustin, Wc=1}
      mask prompts: Zeros "Zeros (enter in s-main:)"; Poles "Poles (enter in s-domain:)"; Gain "Gain (enter in s-domain:)"; AbsTol "Absolute tolerance:"; SampleTime "Sample time:"; Wc "Critical Frequency (Hz):"
      mask help: Continuous mask uses c2d to transform parameters onto the Discrete Zero-Pole block inside.
      mask init: same as ReplayPosFilter/Subsystem/2 FIlter Blend1/1D Filter/Filter2
      mask StyleString: edit,edit,edit,edit,edit,popup(zoh|foh|tustin|prewarp|matched),edit
      mask CallbackString: |||||hidecrit|
      mask Display:
      | droots(zeross,poless,gainss)
      | text( 0.5, 1.0, method, 'verticalAlignment','top')
  "[80k - 120k]" : Saturate  UpperLimit=120000  LowerLimit=80000
  Baro (Gnd) : Outport
  wires:
  Baro (Pa)/1 -> Data Type Conversion/1
  Low Pass8/1(Out1) -> Data Type Conversion1/1
  Data Type Conversion/1 -> Low Pass8/1(In1)
  Data Type Conversion1/1 -> "[80k - 120k]"/1
  "[80k - 120k]"/1 -> Baro (Gnd)/1

== system ReplayPosFilter/Subsystem1/Baro Altimeter/Zero Out Height ==
  Base Height : Inport
  Computed Height : Inport  Port=2
  Enable : EnablePort
  Integer Delay : Delay  DelayLength=1  InitialCondition=0  InputProcessing=Inherited  SampleTime=.01
  Sum : Sum  Inputs=|+-  OutDataTypeStr=single
  Height Offset : Outport
  wires:
  Computed Height/1 -> Integer Delay/1
  Sum/1 -> Height Offset/1
  Integer Delay/1 -> Sum/2
  Base Height/1 -> Sum/1

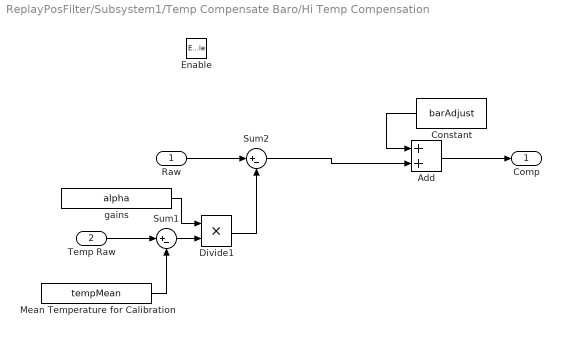
== system ReplayPosFilter/Subsystem1/Temp Compensate Baro/Hi Temp Compensation ==
  Raw : Inport
  Temp Raw : Inport  Port=2
  Enable : EnablePort
  Add : Sum  OutDataTypeStr=single
  Constant : Constant  Value=barAdjust  OutDataTypeStr=single
  Divide1 : Product  OutDataTypeStr=single
  Mean Temperature for Calibration : Constant  Value=tempMean  OutDataTypeStr=single
  Sum1 : Sum  Inputs=|+-  OutDataTypeStr=single
  Sum2 : Sum  Inputs=|+-  OutDataTypeStr=single
  gains : Constant  Value=alpha  OutDataTypeStr=single
  Comp : Outport
  wires:
  Sum2/1 -> Add/2
  Add/1 -> Comp/1
  Constant/1 -> Add/1
  Divide1/1 -> Sum2/2
  gains/1 -> Divide1/1
  Sum1/1 -> Divide1/2
  Temp Raw/1 -> Sum1/1
  Raw/1 -> Sum2/1
  Mean Temperature for Calibration/1 -> Sum1/2

== system ReplayPosFilter/Subsystem1/Temp Compensate Baro/Lo Temp Compensation ==
  Raw : Inport
  Temp Raw : Inport  Port=2
  Enable : EnablePort
  Divide1 : Product  OutDataTypeStr=single
  Mean Temperature for Calibration : Constant  Value=tempMean  OutDataTypeStr=single
  Sum1 : Sum  Inputs=|+-  OutDataTypeStr=single
  Sum2 : Sum  Inputs=|+-  OutDataTypeStr=single
  gains : Constant  Value=alpha  OutDataTypeStr=single
  Comp : Outport
  wires:
  Mean Temperature for Calibration/1 -> Sum1/2
  Raw/1 -> Sum2/1
  Temp Raw/1 -> Sum1/1
  Sum1/1 -> Divide1/2
  gains/1 -> Divide1/1
  Divide1/1 -> Sum2/2
  Sum2/1 -> Comp/1

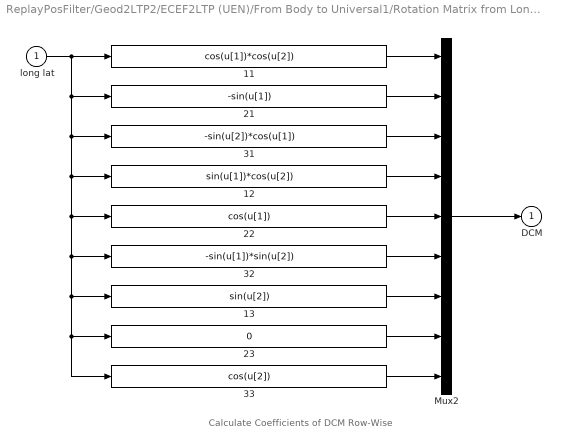
== system ReplayPosFilter/Geod2LTP2/ECEF2LTP (UEN)/From Body to Universal1/Rotation Matrix from Long//Lat ==
  note: Calculate Coefficients of DCM Row-Wise
  long lat : Inport
  11 : Fcn  Expr=cos(u[1])*cos(u[2])
  12 : Fcn  Expr=sin(u[1])*cos(u[2])
  13 : Fcn  Expr=sin(u[2])
  21 : Fcn  Expr=-sin(u[1])
  22 : Fcn  Expr=cos(u[1])
  23 : Fcn  Expr=0
  31 : Fcn  Expr=-sin(u[2])*cos(u[1])
  32 : Fcn  Expr=-sin(u[1])*sin(u[2])
  33 : Fcn  Expr=cos(u[2])
  Mux2 : Mux  Inputs=9
  DCM : Outport
  wires:
  long lat/1 -> 21/1, 31/1, 12/1, 22/1, 32/1, 13/1, 23/1, 33/1, 11/1
  Mux2/1 -> DCM/1
  11/1 -> Mux2/1
  21/1 -> Mux2/2
  31/1 -> Mux2/3
  12/1 -> Mux2/4
  22/1 -> Mux2/5
  32/1 -> Mux2/6
  13/1 -> Mux2/7
  23/1 -> Mux2/8
  33/1 -> Mux2/9

== system ReplayPosFilter/Subsystem/2 FIlter Blend1/1D Filter/Filter2 ==
  In1 : Inport
  Discrete Zero-Pole : DiscreteZeroPole  Zeros=zerosd  Poles=polesd  Gain=gaind  SampleTime=SampleTime
  Out1 : Outport
  wires:
  Discrete Zero-Pole/1 -> Out1/1
  In1/1 -> Discrete Zero-Pole/1

== system ReplayPosFilter/Subsystem/2 FIlter Blend1/1D Filter1/Filter2 ==
  In1 : Inport
  Discrete Zero-Pole : DiscreteZeroPole  Zeros=zerosd  Poles=polesd  Gain=gaind  SampleTime=SampleTime
  Out1 : Outport
  wires:
  In1/1 -> Discrete Zero-Pole/1
  Discrete Zero-Pole/1 -> Out1/1

== system ReplayPosFilter/Subsystem1/Baro Altimeter/Initial Baro Bias/Low Pass8 ==
  In1 : Inport
  Discrete Zero-Pole : DiscreteZeroPole  Zeros=zerosd  Poles=polesd  Gain=gaind  SampleTime=SampleTime
  Out1 : Outport
  wires:
  In1/1 -> Discrete Zero-Pole/1
  Discrete Zero-Pole/1 -> Out1/1

== matlab function Subsystem/2 FIlter Blend1/Embedded MATLAB Function3 ==
  data: gps_h input double size=1; h_rate output double size=1; NewGPS input double size=1; apSampleTime parameter double size=1; baseHeight input double
function h_rate = heightRateAid(gps_h,NewGPS,apSampleTime, baseHeight)
persistent lastGps_h;
persistent TimeSinceLast;
persistent rate;
% persistent lastH;

if (isempty(lastGps_h))
    lastGps_h       = single(0.0);
    TimeSinceLast   = single(apSampleTime);
    rate            = single(0);
%     lastH           = single(-baseHeight);
%     h_rate          = single(0);
end

if (NewGPS)
    rate = single((gps_h - lastGps_h)/TimeSinceLast);
    TimeSinceLast = single(0);
    if (rate > -10.6) && (rate < 17.67)
%         h = lastH + gps_h - lastGps_h;
        h_rate = rate;
    else
%         h = lastH;
        h_rate = single(0);
    end
    lastGps_h = gps_h;
else
%     h = lastH;
    h_rate = single(0);
end

TimeSinceLast = TimeSinceLast + apSampleTime;
% lastH = h;
%%%%%%%%%%%%%%%%%%%%%%%%%%%%%%%%%%%%%%%%%%%%%%%%%%%%%%%%%%%%5
% persistent lastGps_h;
% persistent TimeSinceLast;
% persistent rate;
% persistent lastH;
% 
% if (isempty(lastGps_h))
%     lastGps_h       = single(0.0);
%     TimeSinceLast   = single(apSampleTime);
%     rate            = single(0);
%     lastH           = single(-baseHeight);
%     h_rate          = single(0);
% end
% 
% if (NewGPS)
%     rate = single((gps_h - lastGps_h)/TimeSinceLast);
%     TimeSinceLast = single(0);
%     if (rate > -10.6) && (rate < 17.67)
%         h = lastH + gps_h - lastGps_h;
% %         h_rate = rate;
%     else
%         h = lastH;
% %         h_rate = single(0);
%     end
%     lastGps_h = gps_h;
% else
%     h = lastH;
% %     h_rate = single(0);
% end
% 
% TimeSinceLast = TimeSinceLast + apSampleTime;
% lastH = h;
